simulink model "SustemTagSnab_and_TagElPrivod_Scope"  (R2022a)
settings: Solver=ode23tb  StartTime=0.0  StopTime=10  MaxStep=1e-4  RelTol=1e-5
model workspace (MAT data in the model file):
  pilse = 69.3372055277
undefined symbols (not defined in the file): CF, Es, Filter, OP, RaLa, ReLe, Rsh0, source, TagPr, Tokivx, TP, TS, UravDvij
libraries: spsSeriesRLCBranchLib x18, spsCurrentMeasurementLib x17, spsControlledVoltageSourceLib x8, spsVoltageMeasurementLib x4, spsMeanLib x2, spsIGBTLib x2, spsDiodeLib x1, spsDCVoltageSourceLib x1, msbUtilities x1, spspowerguiLib x1
settings Model: ParameterArgumentNames=pilse  Creator=админ  LastModifiedBy=админ

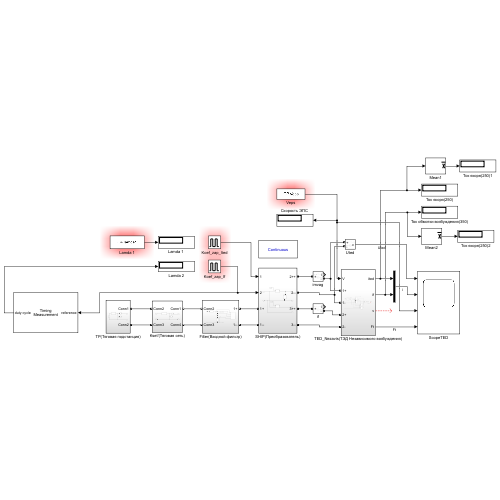
[thumbnail: Simulink's stored preview of the top-level diagram]
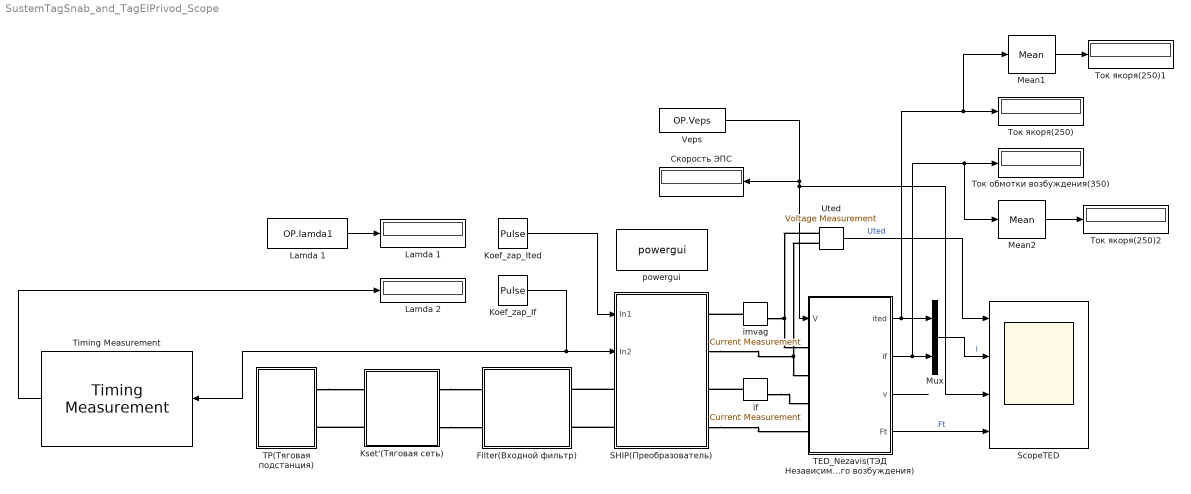
== system SustemTagSnab_and_TagElPrivod_Scope ==
  Filter(Входной фильтр) : Subsystem
  Koef_zap_If : DiscretePulseGenerator  PulseType=Time based  Period=1/source.f_c  PulseWidth=OP.lamda2*100
  Koef_zap_Ited : DiscretePulseGenerator  PulseType=Time based  Period=1/source.f_c  PulseWidth=OP.lamda1*100
  Kset'(Тяговая сеть) : Subsystem
  Lamda 1 : Constant  Value=OP.lamda1
  "Lamda 1 " : Display
  Lamda 2 : Display
      settings: Decimation=3
  Mean1 : spsMeanLib/Mean  Freq=70  Vinit=0  Ts=0
  Mean2 : spsMeanLib/Mean  Freq=70  Vinit=0  Ts=0
  Mux : Mux  Inputs=2
  SHIP(Преобразователь) : Subsystem
  ScopeTED : Scope  NumInputPorts=4
  TED_Nezavis(ТЭД Независимого возбуждения) : Subsystem
  TP(Тяговая подстанция) : Subsystem
  Timing Measurement : msbUtilities/Timing Measurement  Period=off  Frequency=off  RiseTime=off  FallTime=off  DutyCycle=on  Delay=off  SameRefThreshold=on  GlobalRefThreshold=0  Range=[-1 1]  MeasurementType=80% / 20%  ThresholdMax=0.6  ThresholdMin=-0.6  DcRefThreshold=0  DelayRefThreshold=0  DelayTstThreshold=0
      settings: SourceProductBaseCode=AM
  Uted : spsVoltageMeasurementLib/Voltage Measurement  PhasorSimulation=off  OutputType=Complex  PSBequivalent=0
  Veps : Constant  Value=OP.Veps
  if : spsCurrentMeasurementLib/Current Measurement  PhasorSimulation=off  OutputType=Complex  PSBequivalent=0
  imvag : spsCurrentMeasurementLib/Current Measurement  PhasorSimulation=off  OutputType=Complex  PSBequivalent=0
  powergui : spspowerguiLib/powergui  Priority=1  SimulationMode=Continuous  SampleTime=50e-6  frequency=60  Iterations=50  frequencyindice=0  Pbase=100e6  ErrMax=1e-4  UnitsV=kV  UnitsW=MW  buscounter=0  FunctionMessages=off  echomessages=off  EnableUseOfTLC=off  CurrentSourceSwitches=off  DisableSnubberDevices=off  DisableRonSwitches=off  DisableVfSwitches=off  DisplayEquations=off  AutomaticDiscreteSolvers=off  SolverType=Tustin/Backward Euler (TBE)  Interpol=off  ExternalGateDelay=off  methode=off  Ts=100  x0status=blocks  SPID=on  SwTol=0  HookPort=off  NonlinearTolerance=1e-4  nMaxIteration=100  ContinueOnMaxIteration=off  RestoreLinks=warning  ResistiveCurrentMeasurement=off  Frange=[0:2:500]  Ylog=off  Xlog=on  ShowGrid=off  save=off  variable=ZData  structure=0  ZoomFFT=off  StartTime=0.0  cycles=1  DisplayStyle=1  fundamental=60  FreqAxis=off  MaxFrequency=1000  frequencyindicesteady=1  RmsSteady=1  display=off
  "Скорость ЭПС " : Display
  Ток обмотки возбуждения(350) : Display
  Ток якоря(250) : Display
  Ток якоря(250)1 : Display
  Ток якоря(250)2 : Display
  wires:
  Koef_zap_If/1 -> Timing Measurement/1, SHIP(Преобразователь)/2(In2)
  Koef_zap_Ited/1 -> SHIP(Преобразователь)/1(In1)
  Uted/1 -> ScopeTED/1  "Uted"
  TED_Nezavis(ТЭД Независимого возбуждения)/4(Ft) -> ScopeTED/4  "Ft"
  TED_Nezavis(ТЭД Независимого возбуждения)/1(ited) -> Mux/1, Mean1/1, Ток якоря(250)/1
  TED_Nezavis(ТЭД Независимого возбуждения)/2(if) -> Mean2/1, Ток обмотки возбуждения(350)/1, Mux/2
  Mux/1 -> ScopeTED/2  "i"
  Veps/1 -> "Скорость ЭПС "/1, ScopeTED/3, TED_Nezavis(ТЭД Независимого возбуждения)/1(V)
  TED_Nezavis(ТЭД Независимого возбуждения)/3(v) -> ?
  Lamda 1/1 -> "Lamda 1 "/1
  Timing Measurement/1 -> Lamda 2/1
  Mean1/1 -> Ток якоря(250)1/1
  Mean2/1 -> Ток якоря(250)2/1
  connections:
  Kset'(Тяговая сеть)/LConn2 -- TP(Тяговая подстанция)/RConn2
  TP(Тяговая подстанция)/RConn1 -- Kset'(Тяговая сеть)/LConn1
  Kset'(Тяговая сеть)/RConn1 -- Filter(Входной фильтр)/LConn1
  Kset'(Тяговая сеть)/RConn2 -- Filter(Входной фильтр)/LConn2
  SHIP(Преобразователь)/LConn2 -- Filter(Входной фильтр)/RConn2
  SHIP(Преобразователь)/LConn1 -- Filter(Входной фильтр)/RConn1
  imvag/LConn1 -- SHIP(Преобразователь)/RConn1
  imvag/RConn1 -- Uted/LConn1 -- TED_Nezavis(ТЭД Независимого возбуждения)/LConn1
  SHIP(Преобразователь)/RConn2 -- Uted/LConn2 -- TED_Nezavis(ТЭД Независимого возбуждения)/LConn2
  if/LConn1 -- SHIP(Преобразователь)/RConn3
  if/RConn1 -- TED_Nezavis(ТЭД Независимого возбуждения)/LConn3
  SHIP(Преобразователь)/RConn4 -- TED_Nezavis(ТЭД Независимого возбуждения)/LConn4

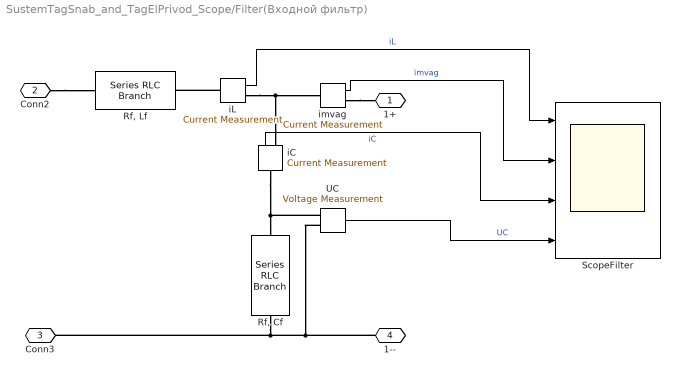
== system SustemTagSnab_and_TagElPrivod_Scope/Filter(Входной фильтр) ==
  "Rf, Cf " : spsSeriesRLCBranchLib/Series RLC Branch  LConnTagsString=__new0  RConnTagsString=__new0  BranchType=RC  Resistance=Filter.R_f  Inductance=1e-3  SetiL0=off  InitialCurrent=0  Capacitance=Filter.C_f  Setx0=off  InitialVoltage=0  Measurements=None
  "Rf, Lf" : spsSeriesRLCBranchLib/Series RLC Branch  LConnTagsString=__new0  RConnTagsString=__new0  BranchType=RL  Resistance=Filter.R_f  Inductance=Filter.L_f  SetiL0=off  InitialCurrent=0  Capacitance=1e-6  Setx0=off  InitialVoltage=0  Measurements=None
  ScopeFilter : Scope  NumInputPorts=4
  UC : spsVoltageMeasurementLib/Voltage Measurement  PhasorSimulation=off  OutputType=Complex  PSBequivalent=0
  iC : spsCurrentMeasurementLib/Current Measurement  PhasorSimulation=off  OutputType=Complex  PSBequivalent=0
  iL : spsCurrentMeasurementLib/Current Measurement  PhasorSimulation=off  OutputType=Complex  PSBequivalent=0
  imvag : spsCurrentMeasurementLib/Current Measurement  PhasorSimulation=off  OutputType=Complex  PSBequivalent=0
  1+ : PMIOPort  Side=Right
  Conn2 : PMIOPort  Port=2  Side=Left
  Conn3 : PMIOPort  Port=3  Side=Left
  1-- : PMIOPort  Port=4  Side=Right
  wires:
  UC/1 -> ScopeFilter/4  "UC"
  iC/1 -> ScopeFilter/3  "iC"
  imvag/1 -> ScopeFilter/2  "imvag"
  iL/1 -> ScopeFilter/1  "iL"
  connections:
  UC/LConn2 -- 1--/RConn1 -- "Rf, Cf "/RConn1 -- Conn3/RConn1
  iC/LConn1 -- UC/LConn1 -- "Rf, Cf "/LConn1
  iL/RConn1 -- imvag/LConn1 -- iC/RConn1
  iL/LConn1 -- "Rf, Lf"/RConn1
  Conn2/RConn1 -- "Rf, Lf"/LConn1
  imvag/RConn1 -- 1+/RConn1

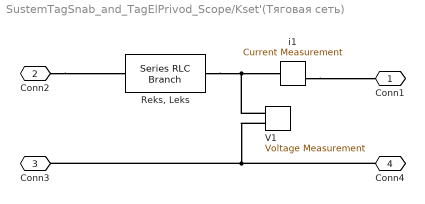
== system SustemTagSnab_and_TagElPrivod_Scope/Kset'(Тяговая сеть) ==
  "Reks, Leks" : spsSeriesRLCBranchLib/Series RLC Branch  LConnTagsString=__new0  RConnTagsString=__new0  BranchType=RL  Resistance=TS.R_eks  Inductance=TS.L_eks  SetiL0=off  InitialCurrent=0  Capacitance=1e-6  Setx0=off  InitialVoltage=0  Measurements=None
  V1 : spsVoltageMeasurementLib/Voltage Measurement  PhasorSimulation=off  OutputType=Complex  PSBequivalent=0
  i1 : spsCurrentMeasurementLib/Current Measurement  PhasorSimulation=off  OutputType=Complex  PSBequivalent=0
  Conn1 : PMIOPort  Side=Right
  Conn2 : PMIOPort  Port=2  Side=Left
  Conn3 : PMIOPort  Port=3  Side=Left
  Conn4 : PMIOPort  Port=4  Side=Right
  connections:
  "Reks, Leks"/RConn1 -- V1/LConn1 -- i1/LConn1
  Conn2/RConn1 -- "Reks, Leks"/LConn1
  i1/RConn1 -- Conn1/RConn1
  V1/LConn2 -- Conn4/RConn1 -- Conn3/RConn1

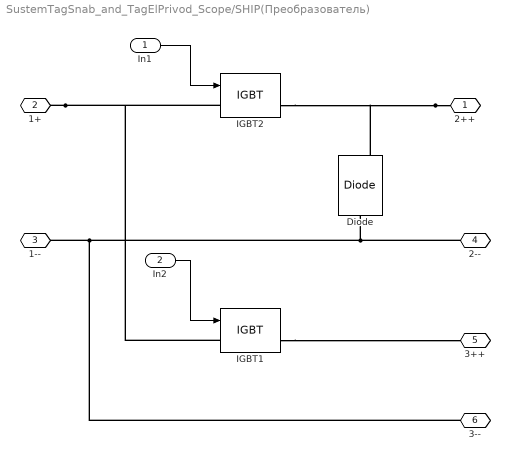
== system SustemTagSnab_and_TagElPrivod_Scope/SHIP(Преобразователь) ==
  In1 : Inport
  In2 : Inport  Port=2
  Diode : spsDiodeLib/Diode  Ron=Diode.r_t  Lon=0  Vf=0.8  IC=0  UseSnubber=0  Rs=Diode.R_s  Cs=250e-9  Measurements=on
  IGBT1 : spsIGBTLib/IGBT  Ron=IGBT.R_on  Lon=0  Vf=IGBT.V_f  Tf=1e-6  Tt=2e-6  IC=0  Rs=1e5  Cs=inf  Measurements=on
  IGBT2 : spsIGBTLib/IGBT  Ron=IGBT.R_on  Lon=0  Vf=IGBT.V_f  Tf=1e-6  Tt=2e-6  IC=0  Rs=1e5  Cs=inf  Measurements=on
  2++ : PMIOPort  Side=Right
  1+ : PMIOPort  Port=2  Side=Left
  1-- : PMIOPort  Port=3  Side=Left
  2-- : PMIOPort  Port=4  Side=Right
  3++ : PMIOPort  Port=5  Side=Right
  3-- : PMIOPort  Port=6  Side=Right
  wires:
  In1/1 -> IGBT2/1
  In2/1 -> IGBT1/1
  connections:
  1+/RConn1 -- IGBT2/LConn1 -- IGBT1/LConn1
  2++/RConn1 -- IGBT2/RConn1 -- Diode/RConn1
  IGBT1/RConn1 -- 3++/RConn1
  2--/RConn1 -- Diode/LConn1 -- 3--/RConn1 -- 1--/RConn1

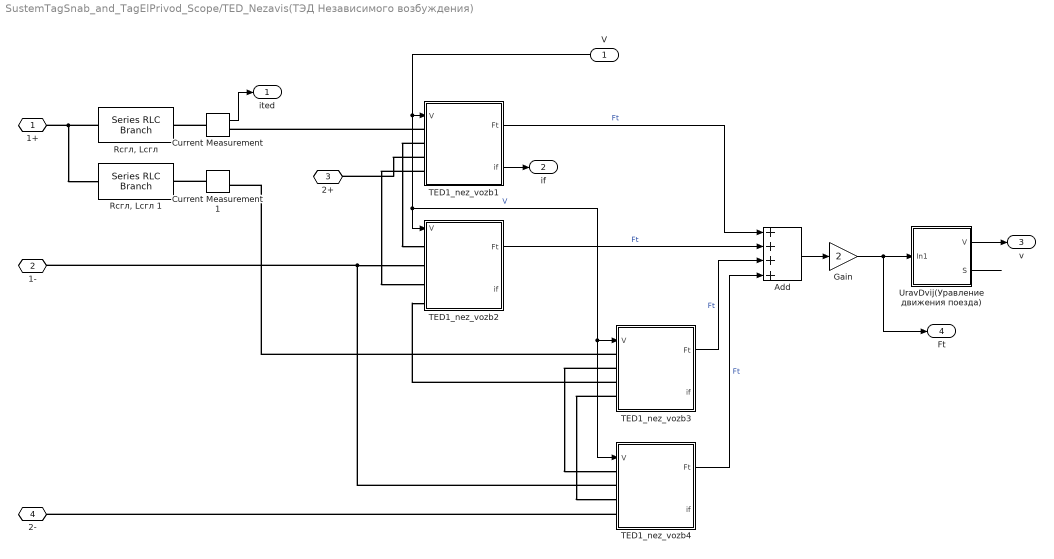
== system SustemTagSnab_and_TagElPrivod_Scope/TED_Nezavis(ТЭД Независимого возбуждения) ==
  V : Inport
  Add : Sum  Inputs=++++
  Current Measurement : spsCurrentMeasurementLib/Current Measurement  PhasorSimulation=off  OutputType=Complex  PSBequivalent=0
  Current Measurement1 : spsCurrentMeasurementLib/Current Measurement  PhasorSimulation=off  OutputType=Complex  PSBequivalent=0
  Gain : Gain  Gain=2
  "Rсгл, Lсгл" : spsSeriesRLCBranchLib/Series RLC Branch  LConnTagsString=__new0  RConnTagsString=__new0  BranchType=RL  Resistance=TagPr.R_sgl  Inductance=TagPr.L_sgl  SetiL0=off  InitialCurrent=0  Capacitance=1e-6  Setx0=off  InitialVoltage=0  Measurements=None
  "Rсгл, Lсгл 1" : spsSeriesRLCBranchLib/Series RLC Branch  LConnTagsString=__new0  RConnTagsString=__new0  BranchType=RL  Resistance=TagPr.R_sgl  Inductance=TagPr.L_sgl  SetiL0=off  InitialCurrent=0  Capacitance=1e-6  Setx0=off  InitialVoltage=0  Measurements=None
  TED1_nez_vozb1 : Subsystem
  TED1_nez_vozb2 : Subsystem
  TED1_nez_vozb3 : Subsystem
  TED1_nez_vozb4 : Subsystem
  UravDvij(Уравление движения поезда) : Subsystem
  1+ : PMIOPort  Side=Left
  1- : PMIOPort  Port=2  Side=Left
  2+ : PMIOPort  Port=3  Side=Left
  2- : PMIOPort  Port=4  Side=Left
  ited : Outport
  if : Outport  Port=2
  v : Outport  Port=3
  Ft : Outport  Port=4
  wires:
  TED1_nez_vozb3/1(Ft) -> Add/3  "Ft"
  TED1_nez_vozb1/1(Ft) -> Add/1  "Ft"
  TED1_nez_vozb2/1(Ft) -> Add/2  "Ft"
  Add/1 -> Gain/1
  TED1_nez_vozb4/1(Ft) -> Add/4  "Ft"
  Gain/1 -> Ft/1, UravDvij(Уравление движения поезда)/1(In1)
  Current Measurement/1 -> ited/1
  TED1_nez_vozb1/2(if) -> if/1
  UravDvij(Уравление движения поезда)/2(S) -> ?
  UravDvij(Уравление движения поезда)/1(V) -> v/1
  V/1 -> TED1_nez_vozb3/1(V), TED1_nez_vozb4/1(V), TED1_nez_vozb2/1(V), TED1_nez_vozb1/1(V)  "V"
  connections:
  TED1_nez_vozb4/LConn2 -- 1-/RConn1 -- TED1_nez_vozb2/LConn2
  TED1_nez_vozb3/LConn2 -- TED1_nez_vozb4/LConn1
  TED1_nez_vozb1/LConn4 -- TED1_nez_vozb2/LConn3
  TED1_nez_vozb1/LConn2 -- TED1_nez_vozb2/LConn1
  "Rсгл, Lсгл"/LConn1 -- "Rсгл, Lсгл 1"/LConn1 -- 1+/RConn1
  TED1_nez_vozb3/LConn3 -- TED1_nez_vozb2/LConn4
  Current Measurement1/LConn1 -- "Rсгл, Lсгл 1"/RConn1
  Current Measurement/LConn1 -- "Rсгл, Lсгл"/RConn1
  TED1_nez_vozb3/LConn1 -- Current Measurement1/RConn1
  TED1_nez_vozb3/LConn4 -- TED1_nez_vozb4/LConn3
  TED1_nez_vozb1/LConn1 -- Current Measurement/RConn1
  TED1_nez_vozb1/LConn3 -- 2+/RConn1
  TED1_nez_vozb4/LConn4 -- 2-/RConn1

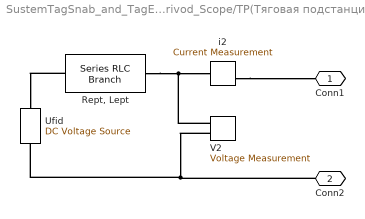
== system SustemTagSnab_and_TagElPrivod_Scope/TP(Тяговая подстанция) ==
  "Rept, Lept" : spsSeriesRLCBranchLib/Series RLC Branch  LConnTagsString=__new0  RConnTagsString=__new0  BranchType=RL  Resistance=TP.R_etp  Inductance=TP.L_etp  SetiL0=off  InitialCurrent=0  Capacitance=1e-6  Setx0=off  InitialVoltage=0  Measurements=None
  Ufid : spsDCVoltageSourceLib/DC Voltage Source  Amplitude=TP.U_tp  Measurements=None
  V2 : spsVoltageMeasurementLib/Voltage Measurement  PhasorSimulation=off  OutputType=Complex  PSBequivalent=0
  i2 : spsCurrentMeasurementLib/Current Measurement  PhasorSimulation=off  OutputType=Complex  PSBequivalent=0
  Conn1 : PMIOPort  Side=Right
  Conn2 : PMIOPort  Port=2  Side=Right
  connections:
  "Rept, Lept"/RConn1 -- V2/LConn1 -- i2/LConn1
  "Rept, Lept"/LConn1 -- Ufid/RConn1
  V2/LConn2 -- Conn2/RConn1 -- Ufid/LConn1
  i2/RConn1 -- Conn1/RConn1

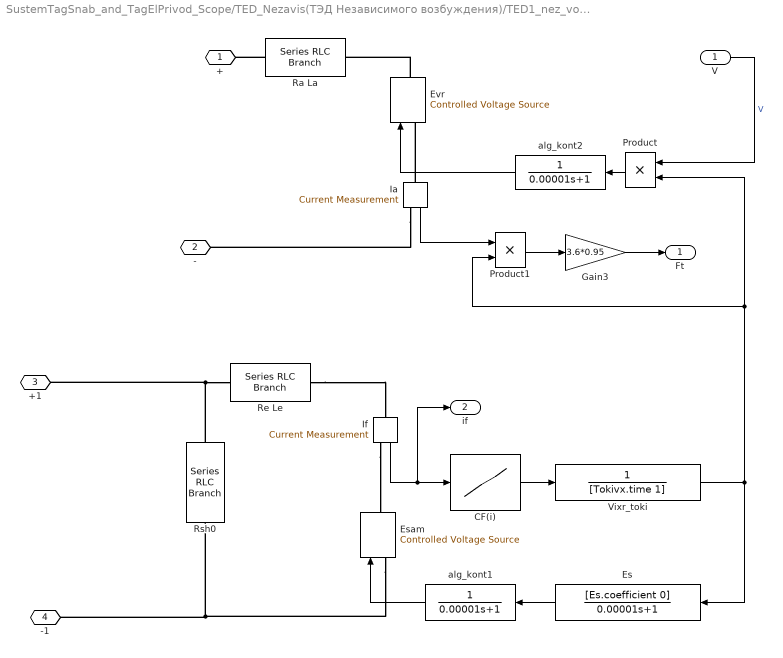
== system SustemTagSnab_and_TagElPrivod_Scope/TED_Nezavis(ТЭД Независимого возбуждения)/TED1_nez_vozb1 ==
  V : Inport
  CF(i) : Lookup_n-D  NumberOfTableDimensions=1  BreakpointsForDimension1=CF.currentvozb  Table=CF.CvF  InternalRulePriority=Speed  RndMeth=Simplest
  Es : TransferFcn  Numerator=[Es.coefficient 0]  Denominator=[0.00001 1]
  Esam : spsControlledVoltageSourceLib/Controlled Voltage Source  Initialize=on  Source_Type=AC  Amplitude=0  Phase=0  Frequency=0  Measurements=None
  Evr : spsControlledVoltageSourceLib/Controlled Voltage Source  Initialize=on  Source_Type=AC  Amplitude=0  Phase=0  Frequency=0  Measurements=None
  Gain3 : Gain  Gain=3.6*0.95
  Ia : spsCurrentMeasurementLib/Current Measurement  PhasorSimulation=off  OutputType=Complex  PSBequivalent=0
  If : spsCurrentMeasurementLib/Current Measurement  PhasorSimulation=off  OutputType=Complex  PSBequivalent=0
  Product : Product
  Product1 : Product
  Ra La : spsSeriesRLCBranchLib/Series RLC Branch  LConnTagsString=__new0  RConnTagsString=__new0  BranchType=RL  Resistance=RaLa.Res  Inductance=RaLa.Ind  SetiL0=off  InitialCurrent=0  Capacitance=1e-6  Setx0=off  InitialVoltage=0  Measurements=None
  Re Le : spsSeriesRLCBranchLib/Series RLC Branch  LConnTagsString=__new0  RConnTagsString=__new0  BranchType=RL  Resistance=ReLe.Res  Inductance=ReLe.Ind  SetiL0=off  InitialCurrent=0  Capacitance=1e-6  Setx0=off  InitialVoltage=0  Measurements=None
  Rsh0 : spsSeriesRLCBranchLib/Series RLC Branch  LConnTagsString=__new0  RConnTagsString=__new0  BranchType=R  Resistance=Rsh0.Res  Inductance=1e-3  SetiL0=off  InitialCurrent=0  Capacitance=1e-6  Setx0=off  InitialVoltage=0  Measurements=None
  Vixr_toki : TransferFcn  Denominator=[Tokivx.time 1]
  alg_kont1 : TransferFcn  Denominator=[0.00001 1]
  alg_kont2 : TransferFcn  Denominator=[0.00001 1]
  + : PMIOPort  Side=Left
  - : PMIOPort  Port=2  Side=Left
  +1 : PMIOPort  Port=3  Side=Left
  -1 : PMIOPort  Port=4  Side=Left
  Ft : Outport
  if : Outport  Port=2
  wires:
  alg_kont2/1 -> Evr/1
  Vixr_toki/1 -> Product1/2, Product/2, Es/1
  Ia/1 -> Product1/1
  Product1/1 -> Gain3/1
  Product/1 -> alg_kont2/1
  Es/1 -> alg_kont1/1
  If/1 -> if/1, CF(i)/1
  alg_kont1/1 -> Esam/1
  CF(i)/1 -> Vixr_toki/1
  V/1 -> Product/1  "V"
  Gain3/1 -> Ft/1
  connections:
  Ia/LConn1 -- Evr/LConn1
  Evr/RConn1 -- Ra La/RConn1
  Rsh0/LConn1 -- +1/RConn1 -- Re Le/LConn1
  If/RConn1 -- Esam/RConn1
  Ia/RConn1 -- -/RConn1
  Esam/LConn1 -- -1/RConn1 -- Rsh0/RConn1
  Re Le/RConn1 -- If/LConn1
  Ra La/LConn1 -- +/RConn1

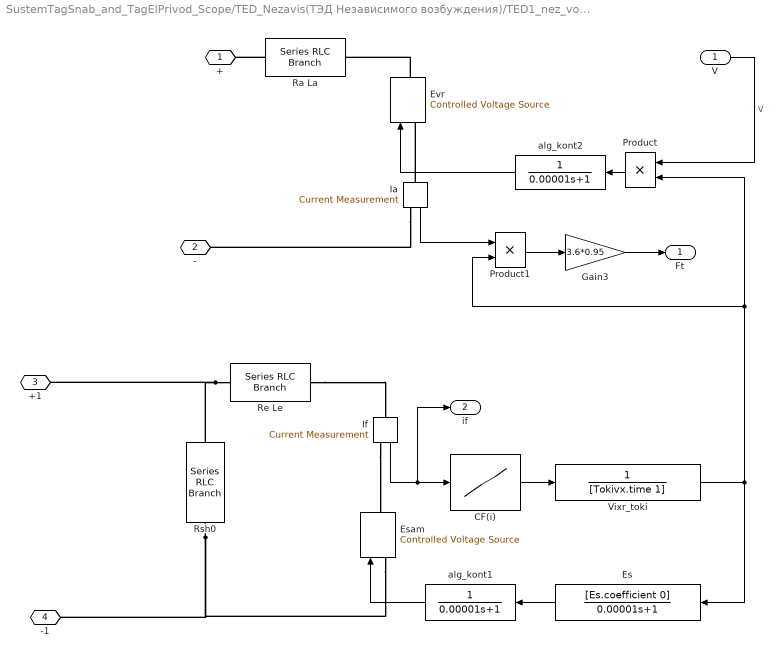
== system SustemTagSnab_and_TagElPrivod_Scope/TED_Nezavis(ТЭД Независимого возбуждения)/TED1_nez_vozb2 ==
  V : Inport
  CF(i) : Lookup_n-D  NumberOfTableDimensions=1  BreakpointsForDimension1=CF.currentvozb  Table=CF.CvF  InternalRulePriority=Speed  RndMeth=Simplest
  Es : TransferFcn  Numerator=[Es.coefficient 0]  Denominator=[0.00001 1]
  Esam : spsControlledVoltageSourceLib/Controlled Voltage Source  Initialize=on  Source_Type=AC  Amplitude=0  Phase=0  Frequency=0  Measurements=None
  Evr : spsControlledVoltageSourceLib/Controlled Voltage Source  Initialize=on  Source_Type=AC  Amplitude=0  Phase=0  Frequency=0  Measurements=None
  Gain3 : Gain  Gain=3.6*0.95
  Ia : spsCurrentMeasurementLib/Current Measurement  PhasorSimulation=off  OutputType=Complex  PSBequivalent=0
  If : spsCurrentMeasurementLib/Current Measurement  PhasorSimulation=off  OutputType=Complex  PSBequivalent=0
  Product : Product
  Product1 : Product
  Ra La : spsSeriesRLCBranchLib/Series RLC Branch  LConnTagsString=__new0  RConnTagsString=__new0  BranchType=RL  Resistance=RaLa.Res  Inductance=RaLa.Ind  SetiL0=off  InitialCurrent=0  Capacitance=1e-6  Setx0=off  InitialVoltage=0  Measurements=None
  Re Le : spsSeriesRLCBranchLib/Series RLC Branch  LConnTagsString=__new0  RConnTagsString=__new0  BranchType=RL  Resistance=ReLe.Res  Inductance=ReLe.Ind  SetiL0=off  InitialCurrent=0  Capacitance=1e-6  Setx0=off  InitialVoltage=0  Measurements=None
  Rsh0 : spsSeriesRLCBranchLib/Series RLC Branch  LConnTagsString=__new0  RConnTagsString=__new0  BranchType=R  Resistance=Rsh0.Res  Inductance=1e-3  SetiL0=off  InitialCurrent=0  Capacitance=1e-6  Setx0=off  InitialVoltage=0  Measurements=None
  Vixr_toki : TransferFcn  Denominator=[Tokivx.time 1]
  alg_kont1 : TransferFcn  Denominator=[0.00001 1]
  alg_kont2 : TransferFcn  Denominator=[0.00001 1]
  + : PMIOPort  Side=Left
  - : PMIOPort  Port=2  Side=Left
  +1 : PMIOPort  Port=3  Side=Left
  -1 : PMIOPort  Port=4  Side=Left
  Ft : Outport
  if : Outport  Port=2
  wires:
  Gain3/1 -> Ft/1
  V/1 -> Product/1  "V"
  CF(i)/1 -> Vixr_toki/1
  alg_kont1/1 -> Esam/1
  If/1 -> CF(i)/1, if/1
  Es/1 -> alg_kont1/1
  Product/1 -> alg_kont2/1
  Product1/1 -> Gain3/1
  Ia/1 -> Product1/1
  Vixr_toki/1 -> Es/1, Product/2, Product1/2
  alg_kont2/1 -> Evr/1
  connections:
  Ra La/LConn1 -- +/RConn1
  Re Le/RConn1 -- If/LConn1
  Rsh0/RConn1 -- -1/RConn1 -- Esam/LConn1
  Ia/RConn1 -- -/RConn1
  If/RConn1 -- Esam/RConn1
  Re Le/LConn1 -- +1/RConn1 -- Rsh0/LConn1
  Evr/RConn1 -- Ra La/RConn1
  Ia/LConn1 -- Evr/LConn1

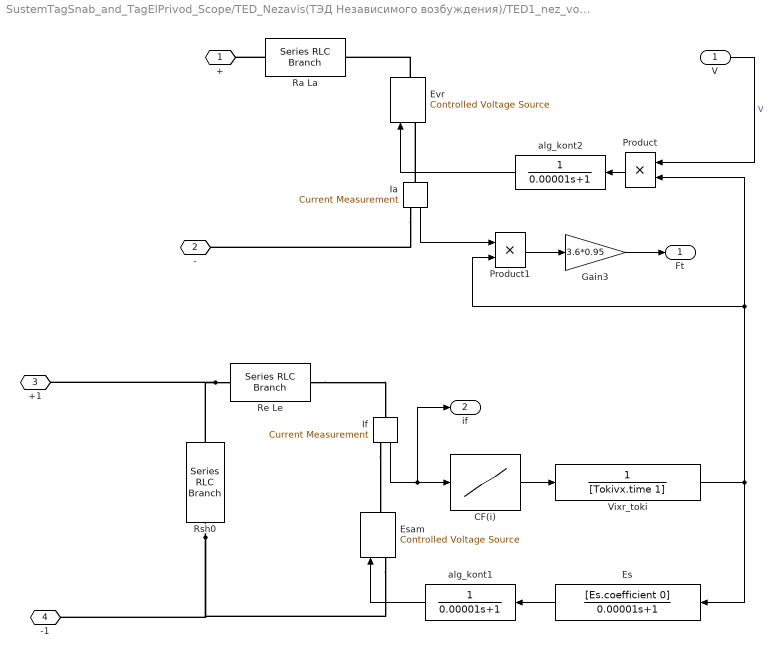
== system SustemTagSnab_and_TagElPrivod_Scope/TED_Nezavis(ТЭД Независимого возбуждения)/TED1_nez_vozb3 ==
  V : Inport
  CF(i) : Lookup_n-D  NumberOfTableDimensions=1  BreakpointsForDimension1=CF.currentvozb  Table=CF.CvF  InternalRulePriority=Speed  RndMeth=Simplest
  Es : TransferFcn  Numerator=[Es.coefficient 0]  Denominator=[0.00001 1]
  Esam : spsControlledVoltageSourceLib/Controlled Voltage Source  Initialize=on  Source_Type=AC  Amplitude=0  Phase=0  Frequency=0  Measurements=None
  Evr : spsControlledVoltageSourceLib/Controlled Voltage Source  Initialize=on  Source_Type=AC  Amplitude=0  Phase=0  Frequency=0  Measurements=None
  Gain3 : Gain  Gain=3.6*0.95
  Ia : spsCurrentMeasurementLib/Current Measurement  PhasorSimulation=off  OutputType=Complex  PSBequivalent=0
  If : spsCurrentMeasurementLib/Current Measurement  PhasorSimulation=off  OutputType=Complex  PSBequivalent=0
  Product : Product
  Product1 : Product
  Ra La : spsSeriesRLCBranchLib/Series RLC Branch  LConnTagsString=__new0  RConnTagsString=__new0  BranchType=RL  Resistance=RaLa.Res  Inductance=RaLa.Ind  SetiL0=off  InitialCurrent=0  Capacitance=1e-6  Setx0=off  InitialVoltage=0  Measurements=None
  Re Le : spsSeriesRLCBranchLib/Series RLC Branch  LConnTagsString=__new0  RConnTagsString=__new0  BranchType=RL  Resistance=ReLe.Res  Inductance=ReLe.Ind  SetiL0=off  InitialCurrent=0  Capacitance=1e-6  Setx0=off  InitialVoltage=0  Measurements=None
  Rsh0 : spsSeriesRLCBranchLib/Series RLC Branch  LConnTagsString=__new0  RConnTagsString=__new0  BranchType=R  Resistance=Rsh0.Res  Inductance=1e-3  SetiL0=off  InitialCurrent=0  Capacitance=1e-6  Setx0=off  InitialVoltage=0  Measurements=None
  Vixr_toki : TransferFcn  Denominator=[Tokivx.time 1]
  alg_kont1 : TransferFcn  Denominator=[0.00001 1]
  alg_kont2 : TransferFcn  Denominator=[0.00001 1]
  + : PMIOPort  Side=Left
  - : PMIOPort  Port=2  Side=Left
  +1 : PMIOPort  Port=3  Side=Left
  -1 : PMIOPort  Port=4  Side=Left
  Ft : Outport
  if : Outport  Port=2
  wires:
  Gain3/1 -> Ft/1
  V/1 -> Product/1  "V"
  CF(i)/1 -> Vixr_toki/1
  alg_kont1/1 -> Esam/1
  If/1 -> CF(i)/1, if/1
  Es/1 -> alg_kont1/1
  Product/1 -> alg_kont2/1
  Product1/1 -> Gain3/1
  Ia/1 -> Product1/1
  Vixr_toki/1 -> Es/1, Product/2, Product1/2
  alg_kont2/1 -> Evr/1
  connections:
  Ra La/LConn1 -- +/RConn1
  Re Le/RConn1 -- If/LConn1
  Rsh0/RConn1 -- -1/RConn1 -- Esam/LConn1
  Ia/RConn1 -- -/RConn1
  If/RConn1 -- Esam/RConn1
  Re Le/LConn1 -- +1/RConn1 -- Rsh0/LConn1
  Evr/RConn1 -- Ra La/RConn1
  Ia/LConn1 -- Evr/LConn1

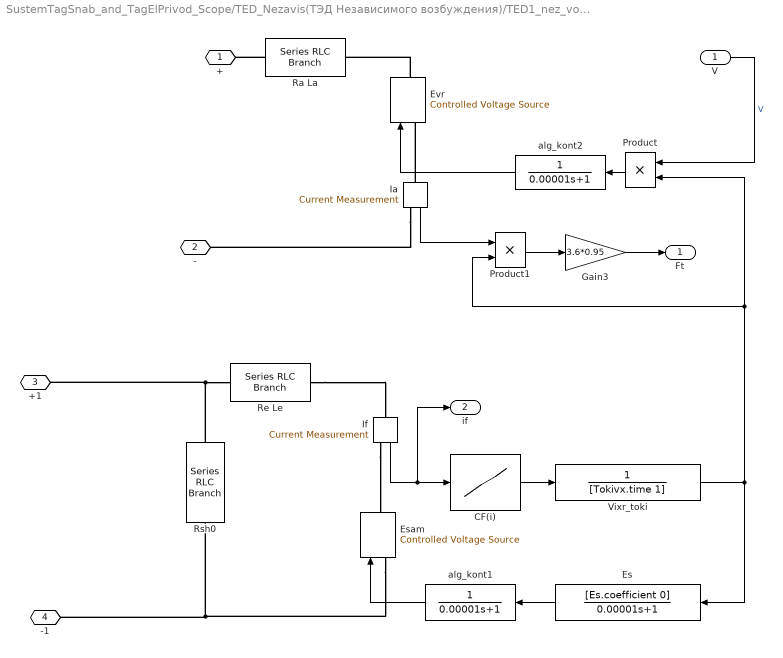
== system SustemTagSnab_and_TagElPrivod_Scope/TED_Nezavis(ТЭД Независимого возбуждения)/TED1_nez_vozb4 ==
  V : Inport
  CF(i) : Lookup_n-D  NumberOfTableDimensions=1  BreakpointsForDimension1=CF.currentvozb  Table=CF.CvF  InternalRulePriority=Speed  RndMeth=Simplest
  Es : TransferFcn  Numerator=[Es.coefficient 0]  Denominator=[0.00001 1]
  Esam : spsControlledVoltageSourceLib/Controlled Voltage Source  Initialize=on  Source_Type=AC  Amplitude=0  Phase=0  Frequency=0  Measurements=None
  Evr : spsControlledVoltageSourceLib/Controlled Voltage Source  Initialize=on  Source_Type=AC  Amplitude=0  Phase=0  Frequency=0  Measurements=None
  Gain3 : Gain  Gain=3.6*0.95
  Ia : spsCurrentMeasurementLib/Current Measurement  PhasorSimulation=off  OutputType=Complex  PSBequivalent=0
  If : spsCurrentMeasurementLib/Current Measurement  PhasorSimulation=off  OutputType=Complex  PSBequivalent=0
  Product : Product
  Product1 : Product
  Ra La : spsSeriesRLCBranchLib/Series RLC Branch  LConnTagsString=__new0  RConnTagsString=__new0  BranchType=RL  Resistance=RaLa.Res  Inductance=RaLa.Ind  SetiL0=off  InitialCurrent=0  Capacitance=1e-6  Setx0=off  InitialVoltage=0  Measurements=None
  Re Le : spsSeriesRLCBranchLib/Series RLC Branch  LConnTagsString=__new0  RConnTagsString=__new0  BranchType=RL  Resistance=ReLe.Res  Inductance=ReLe.Ind  SetiL0=off  InitialCurrent=0  Capacitance=1e-6  Setx0=off  InitialVoltage=0  Measurements=None
  Rsh0 : spsSeriesRLCBranchLib/Series RLC Branch  LConnTagsString=__new0  RConnTagsString=__new0  BranchType=R  Resistance=Rsh0.Res  Inductance=1e-3  SetiL0=off  InitialCurrent=0  Capacitance=1e-6  Setx0=off  InitialVoltage=0  Measurements=None
  Vixr_toki : TransferFcn  Denominator=[Tokivx.time 1]
  alg_kont1 : TransferFcn  Denominator=[0.00001 1]
  alg_kont2 : TransferFcn  Denominator=[0.00001 1]
  + : PMIOPort  Side=Left
  - : PMIOPort  Port=2  Side=Left
  +1 : PMIOPort  Port=3  Side=Left
  -1 : PMIOPort  Port=4  Side=Left
  Ft : Outport
  if : Outport  Port=2
  wires:
  alg_kont2/1 -> Evr/1
  Vixr_toki/1 -> Product1/2, Product/2, Es/1
  Ia/1 -> Product1/1
  Product1/1 -> Gain3/1
  Product/1 -> alg_kont2/1
  Es/1 -> alg_kont1/1
  If/1 -> if/1, CF(i)/1
  alg_kont1/1 -> Esam/1
  CF(i)/1 -> Vixr_toki/1
  V/1 -> Product/1  "V"
  Gain3/1 -> Ft/1
  connections:
  Ia/LConn1 -- Evr/LConn1
  Evr/RConn1 -- Ra La/RConn1
  Rsh0/LConn1 -- +1/RConn1 -- Re Le/LConn1
  If/RConn1 -- Esam/RConn1
  Ia/RConn1 -- -/RConn1
  Esam/LConn1 -- -1/RConn1 -- Rsh0/RConn1
  Re Le/RConn1 -- If/LConn1
  Ra La/LConn1 -- +/RConn1

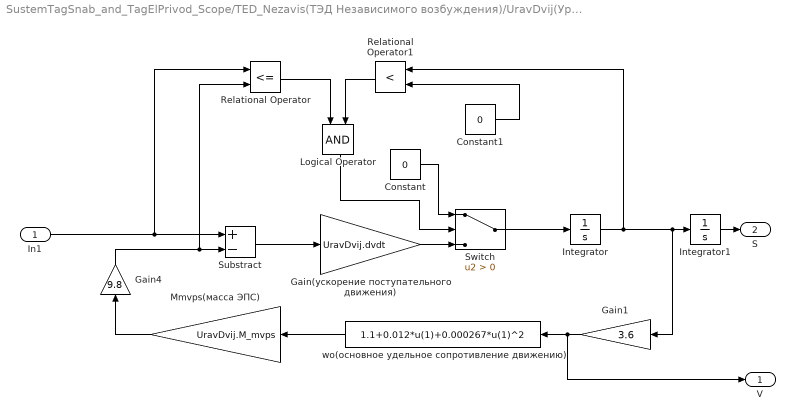
== system SustemTagSnab_and_TagElPrivod_Scope/TED_Nezavis(ТЭД Независимого возбуждения)/UravDvij(Уравление движения поезда) ==
  In1 : Inport
  Constant : Constant  Value=0
  Constant1 : Constant  Value=0
  Gain(ускорение поступательного движения) : Gain  Gain=UravDvij.dvdt
  Gain1 : Gain  Gain=3.6
  Gain4 : Gain  Gain=9.8
  Integrator : Integrator
  Integrator1 : Integrator
  Logical Operator : Logic  AllPortsSameDT=off  OutDataTypeStr=boolean
  Mmvps(масса ЭПС) : Gain  Gain=UravDvij.M_mvps
  Relational Operator : RelationalOperator  Operator=<=  OutDataTypeStr=boolean  RndMeth=Simplest  InputSameDT=off
  Relational Operator1 : RelationalOperator  Operator=<  OutDataTypeStr=boolean  RndMeth=Simplest  InputSameDT=off
  Substract : Sum  Inputs=+-
  Switch : Switch  Criteria=u2 > Threshold  SaturateOnIntegerOverflow=off  InputSameDT=off
  wo(основное удельное сопротивление движению) : Fcn  Expr=1.1+0.012*u(1)+0.000267*u(1)^2
  V : Outport
  S : Outport  Port=2
  wires:
  Switch/1 -> Integrator/1
  wo(основное удельное сопротивление движению)/1 -> Mmvps(масса ЭПС)/1
  Integrator/1 -> Relational Operator1/1, Gain1/1, Integrator1/1
  Gain4/1 -> Relational Operator/2, Substract/2
  Gain1/1 -> V/1, wo(основное удельное сопротивление движению)/1
  In1/1 -> Relational Operator/1, Substract/1
  Constant/1 -> Switch/1
  Relational Operator1/1 -> Logical Operator/2
  Gain(ускорение поступательного движения)/1 -> Switch/3
  Relational Operator/1 -> Logical Operator/1
  Substract/1 -> Gain(ускорение поступательного движения)/1
  Constant1/1 -> Relational Operator1/2
  Logical Operator/1 -> Switch/2
  Integrator1/1 -> S/1
  Mmvps(масса ЭПС)/1 -> Gain4/1
